simulink model "boundingbox2"  (R2018a)
settings: Solver=VariableStepAuto  StartTime=0.0  StopTime=10.0  RelTol=1e-3
libraries: simulink x127
(part 1 of 4)
settings Model: Creator=Rafael  LastModifiedBy=Rafael

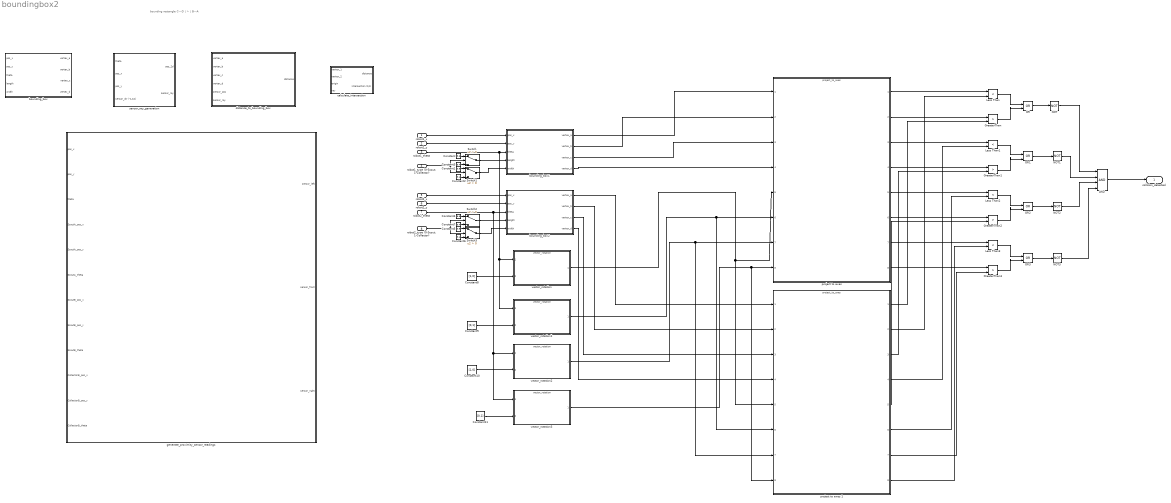
== system boundingbox2 ==
  note: bounding rectangle
      | C---D
      | | > |
      | B---A
  robot1_x : Inport
  robot1_y : Inport  Port=2
  robot1_theta : Inport  Port=3
  robot1_type (0-Scout; 1-Collector) : Inport  Port=4
  robot2_x : Inport  Port=5
  robot2_y : Inport  Port=6
  robot2_theta : Inport  Port=7
  robot2_type (0-Scout; 1-Collector) : Inport  Port=8
  AND : Logic  Inputs=4  IconShape=distinctive  AllPortsSameDT=off  OutDataTypeStr=boolean
  Constant : Constant  Value=8.6
  Constant1 : Constant  Value=9.8
  Constant10 : Constant  Value=[1,0]
  Constant11 : Constant  Value=[0,1]
  Constant{2..3,6..7} (4 alike) : Constant  Value=9.4
  Constant4 : Constant  Value=8.6
  Constant5 : Constant  Value=9.8
  Constant8 : Constant  Value=[1,0]
  Constant9 : Constant  Value=[0,1]
  GreaterThan{,1..3} (4 alike) : RelationalOperator  Operator=>  OutDataTypeStr=boolean  ZeroCross=off  RndMeth=Simplest
  Less Than{,1..3} (4 alike) : RelationalOperator  Operator=<  OutDataTypeStr=boolean  ZeroCross=off  RndMeth=Simplest
  NOT{,1..3} (4 alike) : Logic  Operator=NOT  IconShape=distinctive  AllPortsSameDT=off  OutDataTypeStr=boolean
  OR{,1..3} (4 alike) : Logic  Operator=OR  IconShape=distinctive  AllPortsSameDT=off  OutDataTypeStr=boolean
  Switch{,1..3} (4 alike) : Switch  Criteria=u2 > Threshold  ZeroCross=off
  bounding_box : Subsystem
  bounding_box1 : Subsystem
  bounding_box2 : Subsystem
  "calculate_intersection " : Subsystem
  distance_to_bounding_box : Subsystem
  generate_proximity_sensor_readings : Subsystem
  "project to axes " : ModelReference  ModelNameDialog=project_to_axes  SimulationMode=Normal  ModelReferenceVersion=1.21
  project to axes 1 : ModelReference  ModelNameDialog=project_to_axes  SimulationMode=Normal  ModelReferenceVersion=1.21
  "sensor_ray_generation " : Subsystem
  vector_rotation{,1..3} (4 alike) : ModelReference  ModelNameDialog=vector_rotation  SimulationMode=Normal  ModelReferenceVersion=1.21
  collision_detected : Outport
  wires:
  robot1_x/1 -> bounding_box1/1(pos_x)
  robot1_y/1 -> bounding_box1/2(pos_y)
  robot1_theta/1 -> bounding_box1/3(theta), vector_rotation1/1, vector_rotation/1
  robot1_type (0-Scout; 1-Collector)/1 -> Switch1/2, Switch/2
  Constant/1 -> Switch/1
  Constant1/1 -> Switch1/1
  Constant2/1 -> Switch1/3
  Constant3/1 -> Switch/3
  Switch/1 -> bounding_box1/4(length)
  Switch1/1 -> bounding_box1/5(width)
  robot2_x/1 -> bounding_box2/1(pos_x)
  robot2_y/1 -> bounding_box2/2(pos_y)
  Constant7/1 -> Switch2/3
  Constant6/1 -> Switch3/3
  Constant5/1 -> Switch3/1
  Constant4/1 -> Switch2/1
  robot2_type (0-Scout; 1-Collector)/1 -> Switch2/2, Switch3/2
  Switch2/1 -> bounding_box2/4(length)
  Switch3/1 -> bounding_box2/5(width)
  Constant8/1 -> vector_rotation/2
  Constant9/1 -> vector_rotation1/2
  Constant11/1 -> vector_rotation3/2
  Constant10/1 -> vector_rotation2/2
  robot2_theta/1 -> bounding_box2/3(theta), vector_rotation3/1, vector_rotation2/1
  bounding_box1/1(vertex_a) -> "project to axes "/1
  bounding_box1/2(vertex_b) -> "project to axes "/2
  bounding_box1/3(vertex_c) -> "project to axes "/3
  bounding_box1/4(vertex_d) -> "project to axes "/4
  vector_rotation/1 -> project to axes 1/5, "project to axes "/5
  vector_rotation1/1 -> project to axes 1/6, "project to axes "/6
  vector_rotation2/1 -> project to axes 1/7, "project to axes "/7
  vector_rotation3/1 -> project to axes 1/8, "project to axes "/8
  bounding_box2/1(vertex_a) -> project to axes 1/1
  bounding_box2/2(vertex_b) -> project to axes 1/2
  bounding_box2/3(vertex_c) -> project to axes 1/3
  bounding_box2/4(vertex_d) -> project to axes 1/4
  "project to axes "/1 -> Less Than/1
  project to axes 1/2 -> Less Than/2
  "project to axes "/2 -> GreaterThan/1
  project to axes 1/1 -> GreaterThan/2
  "project to axes "/3 -> Less Than1/1
  project to axes 1/4 -> Less Than1/2
  "project to axes "/4 -> GreaterThan1/1
  project to axes 1/3 -> GreaterThan1/2
  "project to axes "/5 -> Less Than2/1
  project to axes 1/6 -> Less Than2/2
  "project to axes "/6 -> GreaterThan2/1
  "project to axes "/7 -> Less Than3/1
  "project to axes "/8 -> GreaterThan3/1
  project to axes 1/5 -> GreaterThan2/2
  project to axes 1/7 -> GreaterThan3/2
  project to axes 1/8 -> Less Than3/2
  Less Than/1 -> OR/1
  GreaterThan/1 -> OR/2
  Less Than1/1 -> OR1/1
  GreaterThan1/1 -> OR1/2
  Less Than2/1 -> OR2/1
  GreaterThan2/1 -> OR2/2
  Less Than3/1 -> OR3/1
  GreaterThan3/1 -> OR3/2
  OR/1 -> NOT/1
  OR1/1 -> NOT1/1
  OR2/1 -> NOT2/1
  OR3/1 -> NOT3/1
  NOT/1 -> AND/1
  NOT1/1 -> AND/2
  NOT2/1 -> AND/3
  NOT3/1 -> AND/4
  AND/1 -> collision_detected/1

== system boundingbox2/bounding_box ==
  note: output verteces of
      | bounding rectangle
      | C---D
      | |  >  |
      | B---A  as 2d vectors
  pos_x : Inport
  pos_y : Inport  Port=2
  theta : Inport  Port=3
  length : Inport  Port=4
  width : Inport  Port=5
  Add : Sum
  Add1 : Sum
  Gain : Gain  Gain=1/2
  Gain1 : Gain  Gain=1/2
  Gain2 : Gain  Gain=-1
  Subtract : Sum  Inputs=+-
  Subtract1 : Sum  Inputs=+-
  Vector Concatenate : Concatenate
  "vector rotation " : Subsystem
  vector rotation 1 : Subsystem
  vertex_a : Outport
  vertex_b : Outport  Port=2
  vertex_c : Outport  Port=3
  vertex_d : Outport  Port=4
  wires:
  width/1 -> Gain1/1
  length/1 -> Gain/1
  pos_x/1 -> Vector Concatenate/1
  pos_y/1 -> Vector Concatenate/2
  theta/1 -> vector rotation 1/1(angle), "vector rotation "/1(angle)
  Gain/1 -> Gain2/1, "vector rotation "/2(x_dir)
  Gain2/1 -> vector rotation 1/2(x_dir)
  Gain1/1 -> vector rotation 1/3(y_dir), "vector rotation "/3(y_dir)
  Vector Concatenate/1 -> Subtract1/1, Add1/1, Subtract/1, Add/1
  "vector rotation "/1("rotated_vector ") -> Subtract/2, Add/2
  vector rotation 1/1("rotated_vector ") -> Subtract1/2, Add1/2
  Add/1 -> vertex_a/1
  Subtract/1 -> vertex_c/1
  Add1/1 -> vertex_b/1
  Subtract1/1 -> vertex_d/1

== system boundingbox2/bounding_box1 ==
  note: output verteces of
      | bounding rectangle
      | C---D
      | |  >  |
      | B---A  as 2d vectors
  pos_x : Inport
  pos_y : Inport  Port=2
  theta : Inport  Port=3
  length : Inport  Port=4
  width : Inport  Port=5
  Add : Sum
  Add1 : Sum
  Gain : Gain  Gain=1/2
  Gain1 : Gain  Gain=1/2
  Gain2 : Gain  Gain=-1
  Subtract : Sum  Inputs=+-
  Subtract1 : Sum  Inputs=+-
  Vector Concatenate : Concatenate
  "vector rotation " : Subsystem
  vector rotation 1 : Subsystem
  vertex_a : Outport
  vertex_b : Outport  Port=2
  vertex_c : Outport  Port=3
  vertex_d : Outport  Port=4
  wires:
  Subtract1/1 -> vertex_d/1
  Add1/1 -> vertex_b/1
  Subtract/1 -> vertex_c/1
  Add/1 -> vertex_a/1
  vector rotation 1/1("rotated_vector ") -> Add1/2, Subtract1/2
  "vector rotation "/1("rotated_vector ") -> Add/2, Subtract/2
  Vector Concatenate/1 -> Add/1, Subtract/1, Add1/1, Subtract1/1
  Gain1/1 -> "vector rotation "/3(y_dir), vector rotation 1/3(y_dir)
  Gain2/1 -> vector rotation 1/2(x_dir)
  Gain/1 -> "vector rotation "/2(x_dir), Gain2/1
  theta/1 -> "vector rotation "/1(angle), vector rotation 1/1(angle)
  pos_y/1 -> Vector Concatenate/2
  pos_x/1 -> Vector Concatenate/1
  length/1 -> Gain/1
  width/1 -> Gain1/1

== system boundingbox2/bounding_box2 ==
  note: output verteces of
      | bounding rectangle
      | C---D
      | |  >  |
      | B---A  as 2d vectors
  pos_x : Inport
  pos_y : Inport  Port=2
  theta : Inport  Port=3
  length : Inport  Port=4
  width : Inport  Port=5
  Add : Sum
  Add1 : Sum
  Gain : Gain  Gain=1/2
  Gain1 : Gain  Gain=1/2
  Gain2 : Gain  Gain=-1
  Subtract : Sum  Inputs=+-
  Subtract1 : Sum  Inputs=+-
  Vector Concatenate : Concatenate
  "vector rotation " : Subsystem
  vector rotation 1 : Subsystem
  vertex_a : Outport
  vertex_b : Outport  Port=2
  vertex_c : Outport  Port=3
  vertex_d : Outport  Port=4
  wires:
  width/1 -> Gain1/1
  length/1 -> Gain/1
  pos_x/1 -> Vector Concatenate/1
  pos_y/1 -> Vector Concatenate/2
  theta/1 -> vector rotation 1/1(angle), "vector rotation "/1(angle)
  Gain/1 -> Gain2/1, "vector rotation "/2(x_dir)
  Gain2/1 -> vector rotation 1/2(x_dir)
  Gain1/1 -> vector rotation 1/3(y_dir), "vector rotation "/3(y_dir)
  Vector Concatenate/1 -> Subtract1/1, Add1/1, Subtract/1, Add/1
  "vector rotation "/1("rotated_vector ") -> Subtract/2, Add/2
  vector rotation 1/1("rotated_vector ") -> Subtract1/2, Add1/2
  Add/1 -> vertex_a/1
  Subtract/1 -> vertex_c/1
  Add1/1 -> vertex_b/1
  Subtract1/1 -> vertex_d/1

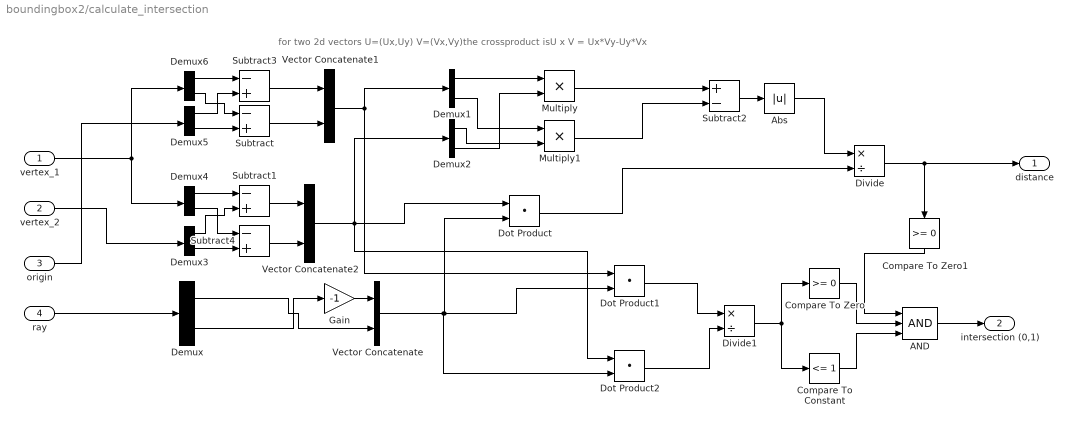
== system boundingbox2/calculate_intersection  ==
  note: for two 2d vectors U=(Ux,Uy) V=(Vx,Vy)the crossproduct isU x V = Ux*Vy-Uy*Vx
  vertex_1 : Inport
  vertex_2 : Inport  Port=2
  "origin " : Inport  Port=3
  ray : Inport  Port=4
  AND : Logic  Inputs=3  IconShape=distinctive  AllPortsSameDT=off  OutDataTypeStr=boolean
  Abs : Abs
  Compare To Constant : simulink/Logic and Bit Operations/Compare To Constant  relop=<=  const=1  OutDataTypeStr=boolean
  Compare To Zero : simulink/Logic and Bit Operations/Compare To Zero  relop=>=  OutDataTypeStr=boolean
  Compare To Zero1 : simulink/Logic and Bit Operations/Compare To Zero  relop=>=  OutDataTypeStr=boolean
  Demux{,1..6} (7 alike) : Demux  Outputs=2
  Divide : Product  Inputs=*/
  Divide1 : Product  Inputs=*/
  Dot Product : DotProduct  InputSameDT=on  OutDataTypeStr=Inherit: Inherit via internal rule
  Dot Product1 : DotProduct  InputSameDT=on  OutDataTypeStr=Inherit: Inherit via internal rule
  Dot Product2 : DotProduct  InputSameDT=on  OutDataTypeStr=Inherit: Inherit via internal rule
  Gain : Gain  Gain=-1
  Multiply : Product
  Multiply1 : Product
  Subtract{,1,3..4} (4 alike) : Sum  Inputs=-+
  Subtract2 : Sum  Inputs=+-
  Vector Concatenate : Concatenate
  Vector Concatenate1 : Concatenate
  Vector Concatenate2 : Concatenate
  distance : Outport
  intersection (0,1) : Outport  Port=2
  wires:
  Compare To Constant/1 -> AND/3
  Compare To Zero/1 -> AND/2
  Divide1/1 -> Compare To Zero/1, Compare To Constant/1
  AND/1 -> intersection (0,1)/1
  Dot Product2/1 -> Divide1/2
  Dot Product1/1 -> Divide1/1
  Multiply1/1 -> Subtract2/2
  Multiply/1 -> Subtract2/1
  Demux2/1 -> Multiply1/2
  Demux1/2 -> Multiply1/1
  Demux2/2 -> Multiply/2
  Demux1/1 -> Multiply/1
  Abs/1 -> Divide/1
  Subtract2/1 -> Abs/1
  Dot Product/1 -> Divide/2
  Divide/1 -> Compare To Zero1/1, distance/1
  Subtract/1 -> Vector Concatenate1/2
  Vector Concatenate/1 -> Dot Product/2, Dot Product1/2, Dot Product2/2
  Demux/1 -> Vector Concatenate/2
  Gain/1 -> Vector Concatenate/1
  Demux/2 -> Gain/1
  ray/1 -> Demux/1
  vertex_2/1 -> Demux3/1
  vertex_1/1 -> Demux6/1, Demux4/1
  "origin "/1 -> Demux5/1
  Demux5/1 -> Subtract3/2
  Demux6/1 -> Subtract3/1
  Demux6/2 -> Subtract/1
  Demux5/2 -> Subtract/2
  Demux4/1 -> Subtract1/1
  Demux4/2 -> Subtract4/1
  Demux3/1 -> Subtract1/2
  Demux3/2 -> Subtract4/2
  Subtract3/1 -> Vector Concatenate1/1
  Vector Concatenate1/1 -> Dot Product1/1, Demux1/1
  Subtract4/1 -> Vector Concatenate2/2
  Subtract1/1 -> Vector Concatenate2/1
  Vector Concatenate2/1 -> Dot Product/1, Demux2/1, Dot Product2/1
  Compare To Zero1/1 -> AND/1

== system boundingbox2/distance_to_bounding_box ==
  note: bounding rectangle
      | C---D
      | |  >  |
      | B---A
  "vertex_a " : Inport
  vertex_b : Inport  Port=2
  vertex_c : Inport  Port=3
  vertex_d : Inport  Port=4
  sensor_pos : Inport  Port=5
  "sensor_ray " : Inport  Port=6
  Inf{,1..3} (4 alike) : Constant  Value=inf
  Min : MinMax  Inputs=4
  Switch{,1..3} (4 alike) : Switch  Criteria=u2 > Threshold
  "calculate_intersection " : Subsystem
  calculate_intersection 1 : Subsystem
  calculate_intersection 2 : Subsystem
  calculate_intersection 3 : Subsystem
  distance : Outport
  wires:
  "vertex_a "/1 -> calculate_intersection 3/2(vertex_2), "calculate_intersection "/1(vertex_1)
  vertex_b/1 -> calculate_intersection 1/1(vertex_1), "calculate_intersection "/2(vertex_2)
  vertex_c/1 -> calculate_intersection 2/1(vertex_1), calculate_intersection 1/2(vertex_2)
  vertex_d/1 -> calculate_intersection 3/1(vertex_1), calculate_intersection 2/2(vertex_2)
  sensor_pos/1 -> calculate_intersection 3/3("origin "), calculate_intersection 2/3("origin "), calculate_intersection 1/3("origin "), "calculate_intersection "/3("origin ")
  "sensor_ray "/1 -> calculate_intersection 3/4(ray), calculate_intersection 2/4(ray), calculate_intersection 1/4(ray), "calculate_intersection "/4(ray)
  "calculate_intersection "/2(intersection (0,1)) -> Switch/2
  Inf/1 -> Switch/3
  Inf1/1 -> Switch1/3
  calculate_intersection 1/2(intersection (0,1)) -> Switch1/2
  calculate_intersection 2/2(intersection (0,1)) -> Switch2/2
  calculate_intersection 3/2(intersection (0,1)) -> Switch3/2
  Inf2/1 -> Switch2/3
  Inf3/1 -> Switch3/3
  calculate_intersection 3/1(distance) -> Switch3/1
  calculate_intersection 2/1(distance) -> Switch2/1
  calculate_intersection 1/1(distance) -> Switch1/1
  "calculate_intersection "/1(distance) -> Switch/1
  Switch/1 -> Min/1
  Switch1/1 -> Min/2
  Switch2/1 -> Min/3
  Switch3/1 -> Min/4
  Min/1 -> distance/1

== system boundingbox2/generate_proximity_sensor_readings ==
  pos_x : Inport
  pos_y : Inport  Port=2
  theta : Inport  Port=3
  ScoutA_pos_x : Inport  Port=4
  ScoutA_pos_y : Inport  Port=5
  ScoutA_theta : Inport  Port=6
  ScoutB_pos_x : Inport  Port=7
  ScoutB_pos_y : Inport  Port=8
  ScoutB_theta : Inport  Port=9
  CollectorB_pos_x : Inport  Port=10
  CollectorB_pos_y : Inport  Port=11
  CollectorB_theta : Inport  Port=12
  Constant{,4..6} (4 alike) : Constant  Value=9.4
  Constant1 : Constant  Value=-1
  Constant2 : Constant  Value=0
  Constant3 : Constant
  Constant7 : Constant  Value=8.6
  Constant8 : Constant  Value=9.8
  Subsystem : Subsystem
  Subsystem1 : Subsystem
  Subsystem2 : Subsystem
  bounding_box_CollectorB : Subsystem
  bounding_box_ScoutA : Subsystem
  bounding_box_ScoutB : Subsystem
  sensor_ray_generation front : Subsystem
  sensor_ray_generation left : Subsystem
  sensor_ray_generation right : Subsystem
  sensor_left : Outport
  sensor_front : Outport  Port=2
  "sensor_right " : Outport  Port=3
  wires:
  theta/1 -> sensor_ray_generation right/1("theta "), sensor_ray_generation front/1("theta "), sensor_ray_generation left/1("theta ")
  bounding_box_CollectorB/2(vertex_b) -> Subsystem2/14(CollectorB_b), Subsystem1/14(CollectorB_b), Subsystem/14(CollectorB_b)
  Constant2/1 -> sensor_ray_generation front/4("sensor_dir (-1,0,1) ")
  Subsystem2/1("sensor_data ") -> "sensor_right "/1
  bounding_box_ScoutB/4(vertex_d) -> Subsystem2/8(ScoutB_d), Subsystem1/8(ScoutB_d), Subsystem/8(ScoutB_d)
  Constant8/1 -> bounding_box_CollectorB/5(width)
  bounding_box_ScoutA/1(vertex_a) -> Subsystem2/5(ScoutA_a), Subsystem1/5(ScoutA_a), Subsystem/5(ScoutA_a)
  bounding_box_CollectorB/3(vertex_c) -> Subsystem2/11(CollectorB_c), Subsystem1/11(CollectorB_c), Subsystem/11(CollectorB_c)
  ScoutB_theta/1 -> bounding_box_ScoutB/3(theta)
  Constant5/1 -> bounding_box_ScoutB/4(length)
  ScoutA_pos_x/1 -> bounding_box_ScoutA/1(pos_x)
  bounding_box_ScoutA/3(vertex_c) -> Subsystem2/3(ScoutA_c), Subsystem1/3(ScoutA_c), Subsystem/3(ScoutA_c)
  Constant6/1 -> bounding_box_ScoutB/5(width)
  Constant1/1 -> sensor_ray_generation left/4("sensor_dir (-1,0,1) ")
  bounding_box_CollectorB/1(vertex_a) -> Subsystem2/13(CollectorB_a), Subsystem1/13(CollectorB_a), Subsystem/13(CollectorB_a)
  bounding_box_ScoutA/4(vertex_d) -> Subsystem2/4(ScoutA_d), Subsystem1/4(ScoutA_d), Subsystem/4(ScoutA_d)
  sensor_ray_generation front/1(pos_2d) -> Subsystem1/1(origin_pos)
  sensor_ray_generation left/2("sensor_ray ") -> Subsystem/2(sensor_ray_dir)
  bounding_box_CollectorB/4(vertex_d) -> Subsystem2/12(CollectorB_d), Subsystem1/12(CollectorB_d), Subsystem/12(CollectorB_d)
  ScoutB_pos_y/1 -> bounding_box_ScoutB/2(pos_y)
  Subsystem/1("sensor_data ") -> sensor_left/1
  pos_y/1 -> sensor_ray_generation left/3(pos_y)
  bounding_box_ScoutB/2(vertex_b) -> Subsystem2/10(ScoutB_b), Subsystem/10(ScoutB_b), Subsystem1/10(ScoutB_b)
  Subsystem1/1("sensor_data ") -> sensor_front/1
  bounding_box_ScoutB/1(vertex_a) -> Subsystem2/9(ScoutB_a), Subsystem1/9(ScoutB_a), Subsystem/9(ScoutB_a)
  bounding_box_ScoutA/2(vertex_b) -> Subsystem2/6(ScoutA_b), Subsystem1/6(ScoutA_b), Subsystem/6(ScoutA_b)
  bounding_box_ScoutB/3(vertex_c) -> Subsystem2/7(ScoutB_c), Subsystem1/7(ScoutB_c), Subsystem/7(ScoutB_c)
  sensor_ray_generation right/2("sensor_ray ") -> Subsystem2/2(sensor_ray_dir)
  ScoutA_pos_y/1 -> bounding_box_ScoutA/2(pos_y)
  CollectorB_theta/1 -> bounding_box_CollectorB/3(theta)
  pos_x/1 -> sensor_ray_generation right/3(pos_y), sensor_ray_generation front/3(pos_y), sensor_ray_generation right/2(pos_x), sensor_ray_generation front/2(pos_x), sensor_ray_generation left/2(pos_x)
  sensor_ray_generation right/1(pos_2d) -> Subsystem2/1(origin_pos)
  Constant4/1 -> bounding_box_ScoutA/5(width)
  CollectorB_pos_x/1 -> bounding_box_CollectorB/1(pos_x)
  Constant/1 -> bounding_box_ScoutA/4(length)
  CollectorB_pos_y/1 -> bounding_box_CollectorB/2(pos_y)
  Constant7/1 -> bounding_box_CollectorB/4(length)
  ScoutA_theta/1 -> bounding_box_ScoutA/3(theta)
  ScoutB_pos_x/1 -> bounding_box_ScoutB/1(pos_x)
  Constant3/1 -> sensor_ray_generation right/4("sensor_dir (-1,0,1) ")
  sensor_ray_generation left/1(pos_2d) -> Subsystem/1(origin_pos)
  sensor_ray_generation front/2("sensor_ray ") -> Subsystem1/2(sensor_ray_dir)

== system boundingbox2/sensor_ray_generation  ==
  "theta " : Inport
  pos_x : Inport  Port=2
  pos_y : Inport  Port=3
  "sensor_dir (-1,0,1) " : Inport  Port=4
  Compare To Zero : simulink/Logic and Bit Operations/Compare To Zero  relop===  OutDataTypeStr=boolean
  Constant : Constant  Value=1.0
  Constant1 : Constant  Value=0
  Switch : Switch  Threshold=1
  Vector Concatenate : Concatenate
  "vector rotation " : Subsystem
  pos_2d : Outport
  "sensor_ray " : Outport  Port=2
  wires:
  "vector rotation "/1("rotated_vector ") -> "sensor_ray "/1
  pos_y/1 -> Vector Concatenate/2
  Vector Concatenate/1 -> pos_2d/1
  pos_x/1 -> Vector Concatenate/1
  "sensor_dir (-1,0,1) "/1 -> Compare To Zero/1, "vector rotation "/3(y_dir)
  "theta "/1 -> "vector rotation "/1(angle)
  Compare To Zero/1 -> Switch/2
  Constant/1 -> Switch/1
  Constant1/1 -> Switch/3
  Switch/1 -> "vector rotation "/2(x_dir)

== system boundingbox2/bounding_box/vector rotation  ==
  angle : Inport
  x_dir : Inport  Port=2
  y_dir : Inport  Port=3
  Cos : Trigonometry  Operator=cos
  Multiply{,1..3} (4 alike) : Product
  Sin : Trigonometry
  Subtract : Sum  Inputs=+-
  Subtract1 : Sum
  Vector Concatenate1 : Concatenate
  "rotated_vector " : Outport
  wires:
  Multiply3/1 -> Subtract1/2
  Multiply1/1 -> Subtract1/1
  Multiply/1 -> Subtract/1
  y_dir/1 -> Multiply3/1, Multiply2/1
  Subtract1/1 -> Vector Concatenate1/2
  Cos/1 -> Multiply3/2, Multiply/2
  Sin/1 -> Multiply1/2, Multiply2/2
  angle/1 -> Cos/1, Sin/1
  x_dir/1 -> Multiply1/1, Multiply/1
  Vector Concatenate1/1 -> "rotated_vector "/1
  Subtract/1 -> Vector Concatenate1/1
  Multiply2/1 -> Subtract/2

== system boundingbox2/bounding_box/vector rotation 1 ==
  angle : Inport
  x_dir : Inport  Port=2
  y_dir : Inport  Port=3
  Cos : Trigonometry  Operator=cos
  Multiply{,1..3} (4 alike) : Product
  Sin : Trigonometry
  Subtract : Sum  Inputs=+-
  Subtract1 : Sum
  Vector Concatenate1 : Concatenate
  "rotated_vector " : Outport
  wires:
  Multiply2/1 -> Subtract/2
  Subtract/1 -> Vector Concatenate1/1
  Vector Concatenate1/1 -> "rotated_vector "/1
  x_dir/1 -> Multiply/1, Multiply1/1
  angle/1 -> Sin/1, Cos/1
  Sin/1 -> Multiply2/2, Multiply1/2
  Cos/1 -> Multiply/2, Multiply3/2
  Subtract1/1 -> Vector Concatenate1/2
  y_dir/1 -> Multiply2/1, Multiply3/1
  Multiply/1 -> Subtract/1
  Multiply1/1 -> Subtract1/1
  Multiply3/1 -> Subtract1/2

== system boundingbox2/bounding_box1/vector rotation  ==
  angle : Inport
  x_dir : Inport  Port=2
  y_dir : Inport  Port=3
  Cos : Trigonometry  Operator=cos
  Multiply{,1..3} (4 alike) : Product
  Sin : Trigonometry
  Subtract : Sum  Inputs=+-
  Subtract1 : Sum
  Vector Concatenate1 : Concatenate
  "rotated_vector " : Outport
  wires:
  Multiply2/1 -> Subtract/2
  Subtract/1 -> Vector Concatenate1/1
  Vector Concatenate1/1 -> "rotated_vector "/1
  x_dir/1 -> Multiply/1, Multiply1/1
  angle/1 -> Sin/1, Cos/1
  Sin/1 -> Multiply2/2, Multiply1/2
  Cos/1 -> Multiply/2, Multiply3/2
  Subtract1/1 -> Vector Concatenate1/2
  y_dir/1 -> Multiply2/1, Multiply3/1
  Multiply/1 -> Subtract/1
  Multiply1/1 -> Subtract1/1
  Multiply3/1 -> Subtract1/2

== system boundingbox2/bounding_box1/vector rotation 1 ==
  angle : Inport
  x_dir : Inport  Port=2
  y_dir : Inport  Port=3
  Cos : Trigonometry  Operator=cos
  Multiply{,1..3} (4 alike) : Product
  Sin : Trigonometry
  Subtract : Sum  Inputs=+-
  Subtract1 : Sum
  Vector Concatenate1 : Concatenate
  "rotated_vector " : Outport
  wires:
  Multiply3/1 -> Subtract1/2
  Multiply1/1 -> Subtract1/1
  Multiply/1 -> Subtract/1
  y_dir/1 -> Multiply3/1, Multiply2/1
  Subtract1/1 -> Vector Concatenate1/2
  Cos/1 -> Multiply3/2, Multiply/2
  Sin/1 -> Multiply1/2, Multiply2/2
  angle/1 -> Cos/1, Sin/1
  x_dir/1 -> Multiply1/1, Multiply/1
  Vector Concatenate1/1 -> "rotated_vector "/1
  Subtract/1 -> Vector Concatenate1/1
  Multiply2/1 -> Subtract/2

== system boundingbox2/bounding_box2/vector rotation  ==
  angle : Inport
  x_dir : Inport  Port=2
  y_dir : Inport  Port=3
  Cos : Trigonometry  Operator=cos
  Multiply{,1..3} (4 alike) : Product
  Sin : Trigonometry
  Subtract : Sum  Inputs=+-
  Subtract1 : Sum
  Vector Concatenate1 : Concatenate
  "rotated_vector " : Outport
  wires:
  Multiply3/1 -> Subtract1/2
  Multiply1/1 -> Subtract1/1
  Multiply/1 -> Subtract/1
  y_dir/1 -> Multiply3/1, Multiply2/1
  Subtract1/1 -> Vector Concatenate1/2
  Cos/1 -> Multiply3/2, Multiply/2
  Sin/1 -> Multiply1/2, Multiply2/2
  angle/1 -> Cos/1, Sin/1
  x_dir/1 -> Multiply1/1, Multiply/1
  Vector Concatenate1/1 -> "rotated_vector "/1
  Subtract/1 -> Vector Concatenate1/1
  Multiply2/1 -> Subtract/2

== system boundingbox2/bounding_box2/vector rotation 1 ==
  angle : Inport
  x_dir : Inport  Port=2
  y_dir : Inport  Port=3
  Cos : Trigonometry  Operator=cos
  Multiply{,1..3} (4 alike) : Product
  Sin : Trigonometry
  Subtract : Sum  Inputs=+-
  Subtract1 : Sum
  Vector Concatenate1 : Concatenate
  "rotated_vector " : Outport
  wires:
  Multiply2/1 -> Subtract/2
  Subtract/1 -> Vector Concatenate1/1
  Vector Concatenate1/1 -> "rotated_vector "/1
  x_dir/1 -> Multiply/1, Multiply1/1
  angle/1 -> Sin/1, Cos/1
  Sin/1 -> Multiply2/2, Multiply1/2
  Cos/1 -> Multiply/2, Multiply3/2
  Subtract1/1 -> Vector Concatenate1/2
  y_dir/1 -> Multiply2/1, Multiply3/1
  Multiply/1 -> Subtract/1
  Multiply1/1 -> Subtract1/1
  Multiply3/1 -> Subtract1/2

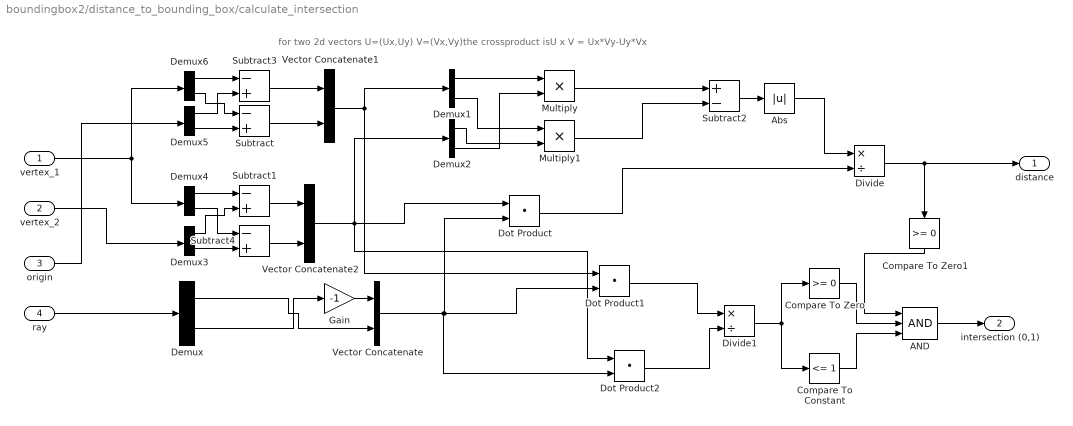
== system boundingbox2/distance_to_bounding_box/calculate_intersection  ==
  note: for two 2d vectors U=(Ux,Uy) V=(Vx,Vy)the crossproduct isU x V = Ux*Vy-Uy*Vx
  vertex_1 : Inport
  vertex_2 : Inport  Port=2
  "origin " : Inport  Port=3
  ray : Inport  Port=4
  AND : Logic  Inputs=3  IconShape=distinctive  AllPortsSameDT=off  OutDataTypeStr=boolean
  Abs : Abs
  Compare To Constant : simulink/Logic and Bit Operations/Compare To Constant  relop=<=  const=1  OutDataTypeStr=boolean
  Compare To Zero : simulink/Logic and Bit Operations/Compare To Zero  relop=>=  OutDataTypeStr=boolean
  Compare To Zero1 : simulink/Logic and Bit Operations/Compare To Zero  relop=>=  OutDataTypeStr=boolean
  Demux{,1..6} (7 alike) : Demux  Outputs=2
  Divide : Product  Inputs=*/
  Divide1 : Product  Inputs=*/
  Dot Product : DotProduct  InputSameDT=on  OutDataTypeStr=Inherit: Inherit via internal rule
  Dot Product1 : DotProduct  InputSameDT=on  OutDataTypeStr=Inherit: Inherit via internal rule
  Dot Product2 : DotProduct  InputSameDT=on  OutDataTypeStr=Inherit: Inherit via internal rule
  Gain : Gain  Gain=-1
  Multiply : Product
  Multiply1 : Product
  Subtract{,1,3..4} (4 alike) : Sum  Inputs=-+
  Subtract2 : Sum  Inputs=+-
  Vector Concatenate : Concatenate
  Vector Concatenate1 : Concatenate
  Vector Concatenate2 : Concatenate
  distance : Outport
  intersection (0,1) : Outport  Port=2
  wires:
  Compare To Constant/1 -> AND/3
  Compare To Zero/1 -> AND/2
  Divide1/1 -> Compare To Zero/1, Compare To Constant/1
  AND/1 -> intersection (0,1)/1
  Dot Product2/1 -> Divide1/2
  Dot Product1/1 -> Divide1/1
  Multiply1/1 -> Subtract2/2
  Multiply/1 -> Subtract2/1
  Demux2/1 -> Multiply1/2
  Demux1/2 -> Multiply1/1
  Demux2/2 -> Multiply/2
  Demux1/1 -> Multiply/1
  Abs/1 -> Divide/1
  Subtract2/1 -> Abs/1
  Dot Product/1 -> Divide/2
  Divide/1 -> Compare To Zero1/1, distance/1
  Subtract/1 -> Vector Concatenate1/2
  Vector Concatenate/1 -> Dot Product/2, Dot Product1/2, Dot Product2/2
  Demux/1 -> Vector Concatenate/2
  Gain/1 -> Vector Concatenate/1
  Demux/2 -> Gain/1
  ray/1 -> Demux/1
  vertex_2/1 -> Demux3/1
  vertex_1/1 -> Demux6/1, Demux4/1
  "origin "/1 -> Demux5/1
  Demux5/1 -> Subtract3/2
  Demux6/1 -> Subtract3/1
  Demux6/2 -> Subtract/1
  Demux5/2 -> Subtract/2
  Demux4/1 -> Subtract1/1
  Demux4/2 -> Subtract4/1
  Demux3/1 -> Subtract1/2
  Demux3/2 -> Subtract4/2
  Subtract3/1 -> Vector Concatenate1/1
  Vector Concatenate1/1 -> Dot Product1/1, Demux1/1
  Subtract4/1 -> Vector Concatenate2/2
  Subtract1/1 -> Vector Concatenate2/1
  Vector Concatenate2/1 -> Dot Product/1, Demux2/1, Dot Product2/1
  Compare To Zero1/1 -> AND/1

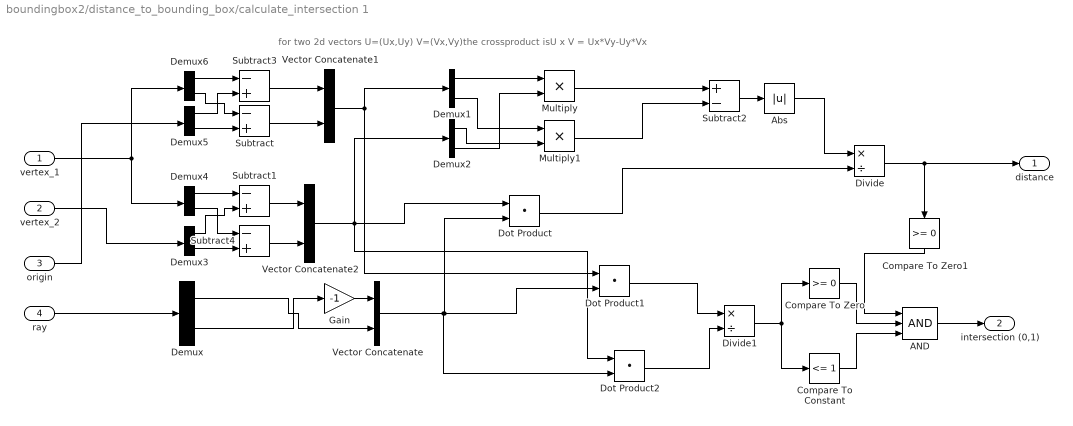
== system boundingbox2/distance_to_bounding_box/calculate_intersection 1 ==
  note: for two 2d vectors U=(Ux,Uy) V=(Vx,Vy)the crossproduct isU x V = Ux*Vy-Uy*Vx
  vertex_1 : Inport
  vertex_2 : Inport  Port=2
  "origin " : Inport  Port=3
  ray : Inport  Port=4
  AND : Logic  Inputs=3  IconShape=distinctive  AllPortsSameDT=off  OutDataTypeStr=boolean
  Abs : Abs
  Compare To Constant : simulink/Logic and Bit Operations/Compare To Constant  relop=<=  const=1  OutDataTypeStr=boolean
  Compare To Zero : simulink/Logic and Bit Operations/Compare To Zero  relop=>=  OutDataTypeStr=boolean
  Compare To Zero1 : simulink/Logic and Bit Operations/Compare To Zero  relop=>=  OutDataTypeStr=boolean
  Demux{,1..6} (7 alike) : Demux  Outputs=2
  Divide : Product  Inputs=*/
  Divide1 : Product  Inputs=*/
  Dot Product : DotProduct  InputSameDT=on  OutDataTypeStr=Inherit: Inherit via internal rule
  Dot Product1 : DotProduct  InputSameDT=on  OutDataTypeStr=Inherit: Inherit via internal rule
  Dot Product2 : DotProduct  InputSameDT=on  OutDataTypeStr=Inherit: Inherit via internal rule
  Gain : Gain  Gain=-1
  Multiply : Product
  Multiply1 : Product
  Subtract{,1,3..4} (4 alike) : Sum  Inputs=-+
  Subtract2 : Sum  Inputs=+-
  Vector Concatenate : Concatenate
  Vector Concatenate1 : Concatenate
  Vector Concatenate2 : Concatenate
  distance : Outport
  intersection (0,1) : Outport  Port=2
  wires:
  Compare To Zero1/1 -> AND/1
  Vector Concatenate2/1 -> Dot Product2/1, Demux2/1, Dot Product/1
  Subtract1/1 -> Vector Concatenate2/1
  Subtract4/1 -> Vector Concatenate2/2
  Vector Concatenate1/1 -> Demux1/1, Dot Product1/1
  Subtract3/1 -> Vector Concatenate1/1
  Demux3/2 -> Subtract4/2
  Demux3/1 -> Subtract1/2
  Demux4/2 -> Subtract4/1
  Demux4/1 -> Subtract1/1
  Demux5/2 -> Subtract/2
  Demux6/2 -> Subtract/1
  Demux6/1 -> Subtract3/1
  Demux5/1 -> Subtract3/2
  "origin "/1 -> Demux5/1
  vertex_1/1 -> Demux4/1, Demux6/1
  vertex_2/1 -> Demux3/1
  ray/1 -> Demux/1
  Demux/2 -> Gain/1
  Gain/1 -> Vector Concatenate/1
  Demux/1 -> Vector Concatenate/2
  Vector Concatenate/1 -> Dot Product2/2, Dot Product1/2, Dot Product/2
  Subtract/1 -> Vector Concatenate1/2
  Divide/1 -> distance/1, Compare To Zero1/1
  Dot Product/1 -> Divide/2
  Subtract2/1 -> Abs/1
  Abs/1 -> Divide/1
  Demux1/1 -> Multiply/1
  Demux2/2 -> Multiply/2
  Demux1/2 -> Multiply1/1
  Demux2/1 -> Multiply1/2
  Multiply/1 -> Subtract2/1
  Multiply1/1 -> Subtract2/2
  Dot Product1/1 -> Divide1/1
  Dot Product2/1 -> Divide1/2
  AND/1 -> intersection (0,1)/1
  Divide1/1 -> Compare To Constant/1, Compare To Zero/1
  Compare To Zero/1 -> AND/2
  Compare To Constant/1 -> AND/3

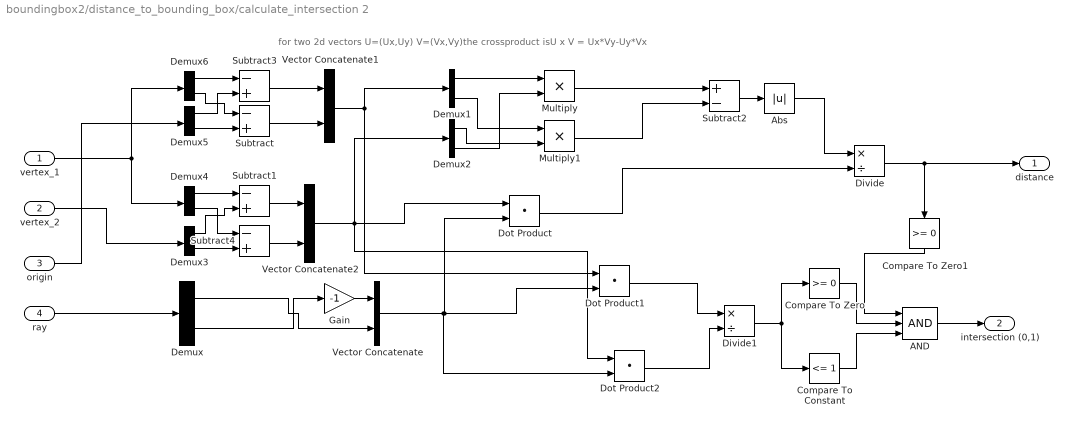
== system boundingbox2/distance_to_bounding_box/calculate_intersection 2 ==
  note: for two 2d vectors U=(Ux,Uy) V=(Vx,Vy)the crossproduct isU x V = Ux*Vy-Uy*Vx
  vertex_1 : Inport
  vertex_2 : Inport  Port=2
  "origin " : Inport  Port=3
  ray : Inport  Port=4
  AND : Logic  Inputs=3  IconShape=distinctive  AllPortsSameDT=off  OutDataTypeStr=boolean
  Abs : Abs
  Compare To Constant : simulink/Logic and Bit Operations/Compare To Constant  relop=<=  const=1  OutDataTypeStr=boolean
  Compare To Zero : simulink/Logic and Bit Operations/Compare To Zero  relop=>=  OutDataTypeStr=boolean
  Compare To Zero1 : simulink/Logic and Bit Operations/Compare To Zero  relop=>=  OutDataTypeStr=boolean
  Demux{,1..6} (7 alike) : Demux  Outputs=2
  Divide : Product  Inputs=*/
  Divide1 : Product  Inputs=*/
  Dot Product : DotProduct  InputSameDT=on  OutDataTypeStr=Inherit: Inherit via internal rule
  Dot Product1 : DotProduct  InputSameDT=on  OutDataTypeStr=Inherit: Inherit via internal rule
  Dot Product2 : DotProduct  InputSameDT=on  OutDataTypeStr=Inherit: Inherit via internal rule
  Gain : Gain  Gain=-1
  Multiply : Product
  Multiply1 : Product
  Subtract{,1,3..4} (4 alike) : Sum  Inputs=-+
  Subtract2 : Sum  Inputs=+-
  Vector Concatenate : Concatenate
  Vector Concatenate1 : Concatenate
  Vector Concatenate2 : Concatenate
  distance : Outport
  intersection (0,1) : Outport  Port=2
  wires:
  Compare To Constant/1 -> AND/3
  Compare To Zero/1 -> AND/2
  Divide1/1 -> Compare To Zero/1, Compare To Constant/1
  AND/1 -> intersection (0,1)/1
  Dot Product2/1 -> Divide1/2
  Dot Product1/1 -> Divide1/1
  Multiply1/1 -> Subtract2/2
  Multiply/1 -> Subtract2/1
  Demux2/1 -> Multiply1/2
  Demux1/2 -> Multiply1/1
  Demux2/2 -> Multiply/2
  Demux1/1 -> Multiply/1
  Abs/1 -> Divide/1
  Subtract2/1 -> Abs/1
  Dot Product/1 -> Divide/2
  Divide/1 -> Compare To Zero1/1, distance/1
  Subtract/1 -> Vector Concatenate1/2
  Vector Concatenate/1 -> Dot Product/2, Dot Product1/2, Dot Product2/2
  Demux/1 -> Vector Concatenate/2
  Gain/1 -> Vector Concatenate/1
  Demux/2 -> Gain/1
  ray/1 -> Demux/1
  vertex_2/1 -> Demux3/1
  vertex_1/1 -> Demux6/1, Demux4/1
  "origin "/1 -> Demux5/1
  Demux5/1 -> Subtract3/2
  Demux6/1 -> Subtract3/1
  Demux6/2 -> Subtract/1
  Demux5/2 -> Subtract/2
  Demux4/1 -> Subtract1/1
  Demux4/2 -> Subtract4/1
  Demux3/1 -> Subtract1/2
  Demux3/2 -> Subtract4/2
  Subtract3/1 -> Vector Concatenate1/1
  Vector Concatenate1/1 -> Dot Product1/1, Demux1/1
  Subtract4/1 -> Vector Concatenate2/2
  Subtract1/1 -> Vector Concatenate2/1
  Vector Concatenate2/1 -> Dot Product/1, Demux2/1, Dot Product2/1
  Compare To Zero1/1 -> AND/1

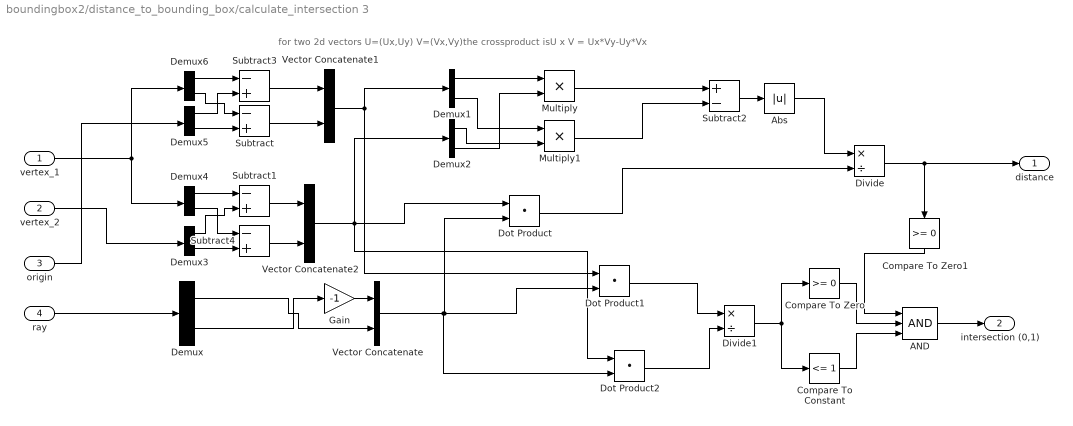
== system boundingbox2/distance_to_bounding_box/calculate_intersection 3 ==
  note: for two 2d vectors U=(Ux,Uy) V=(Vx,Vy)the crossproduct isU x V = Ux*Vy-Uy*Vx
  vertex_1 : Inport
  vertex_2 : Inport  Port=2
  "origin " : Inport  Port=3
  ray : Inport  Port=4
  AND : Logic  Inputs=3  IconShape=distinctive  AllPortsSameDT=off  OutDataTypeStr=boolean
  Abs : Abs
  Compare To Constant : simulink/Logic and Bit Operations/Compare To Constant  relop=<=  const=1  OutDataTypeStr=boolean
  Compare To Zero : simulink/Logic and Bit Operations/Compare To Zero  relop=>=  OutDataTypeStr=boolean
  Compare To Zero1 : simulink/Logic and Bit Operations/Compare To Zero  relop=>=  OutDataTypeStr=boolean
  Demux{,1..6} (7 alike) : Demux  Outputs=2
  Divide : Product  Inputs=*/
  Divide1 : Product  Inputs=*/
  Dot Product : DotProduct  InputSameDT=on  OutDataTypeStr=Inherit: Inherit via internal rule
  Dot Product1 : DotProduct  InputSameDT=on  OutDataTypeStr=Inherit: Inherit via internal rule
  Dot Product2 : DotProduct  InputSameDT=on  OutDataTypeStr=Inherit: Inherit via internal rule
  Gain : Gain  Gain=-1
  Multiply : Product
  Multiply1 : Product
  Subtract{,1,3..4} (4 alike) : Sum  Inputs=-+
  Subtract2 : Sum  Inputs=+-
  Vector Concatenate : Concatenate
  Vector Concatenate1 : Concatenate
  Vector Concatenate2 : Concatenate
  distance : Outport
  intersection (0,1) : Outport  Port=2
  wires:
  Compare To Zero1/1 -> AND/1
  Vector Concatenate2/1 -> Dot Product2/1, Demux2/1, Dot Product/1
  Subtract1/1 -> Vector Concatenate2/1
  Subtract4/1 -> Vector Concatenate2/2
  Vector Concatenate1/1 -> Demux1/1, Dot Product1/1
  Subtract3/1 -> Vector Concatenate1/1
  Demux3/2 -> Subtract4/2
  Demux3/1 -> Subtract1/2
  Demux4/2 -> Subtract4/1
  Demux4/1 -> Subtract1/1
  Demux5/2 -> Subtract/2
  Demux6/2 -> Subtract/1
  Demux6/1 -> Subtract3/1
  Demux5/1 -> Subtract3/2
  "origin "/1 -> Demux5/1
  vertex_1/1 -> Demux4/1, Demux6/1
  vertex_2/1 -> Demux3/1
  ray/1 -> Demux/1
  Demux/2 -> Gain/1
  Gain/1 -> Vector Concatenate/1
  Demux/1 -> Vector Concatenate/2
  Vector Concatenate/1 -> Dot Product2/2, Dot Product1/2, Dot Product/2
  Subtract/1 -> Vector Concatenate1/2
  Divide/1 -> distance/1, Compare To Zero1/1
  Dot Product/1 -> Divide/2
  Subtract2/1 -> Abs/1
  Abs/1 -> Divide/1
  Demux1/1 -> Multiply/1
  Demux2/2 -> Multiply/2
  Demux1/2 -> Multiply1/1
  Demux2/1 -> Multiply1/2
  Multiply/1 -> Subtract2/1
  Multiply1/1 -> Subtract2/2
  Dot Product1/1 -> Divide1/1
  Dot Product2/1 -> Divide1/2
  AND/1 -> intersection (0,1)/1
  Divide1/1 -> Compare To Constant/1, Compare To Zero/1
  Compare To Zero/1 -> AND/2
  Compare To Constant/1 -> AND/3

== system boundingbox2/generate_proximity_sensor_readings/Subsystem ==
  origin_pos : Inport
  sensor_ray_dir : Inport  Port=2
  ScoutA_c : Inport  Port=3
  ScoutA_d : Inport  Port=4
  ScoutA_a : Inport  Port=5
  ScoutA_b : Inport  Port=6
  ScoutB_c : Inport  Port=7
  ScoutB_d : Inport  Port=8
  ScoutB_a : Inport  Port=9
  ScoutB_b : Inport  Port=10
  CollectorB_c : Inport  Port=11
  CollectorB_d : Inport  Port=12
  CollectorB_a : Inport  Port=13
  CollectorB_b : Inport  Port=14
  Min : MinMax  Inputs=3
  distance_to_bounding_box : Subsystem
  distance_to_bounding_box1 : Subsystem
  distance_to_bounding_box2 : Subsystem
  "distance_to_proximity_sensor_data " : Subsystem
  "sensor_data " : Outport
  wires:
  distance_to_bounding_box/1(distance) -> Min/1
  sensor_ray_dir/1 -> distance_to_bounding_box/6("sensor_ray "), distance_to_bounding_box1/6("sensor_ray "), distance_to_bounding_box2/6("sensor_ray ")
  Min/1 -> "distance_to_proximity_sensor_data "/1(distance_cm)
  origin_pos/1 -> distance_to_bounding_box/5(sensor_pos), distance_to_bounding_box1/5(sensor_pos), distance_to_bounding_box2/5(sensor_pos)
  ScoutA_c/1 -> distance_to_bounding_box/3(vertex_c)
  ScoutA_b/1 -> distance_to_bounding_box/2(vertex_b)
  CollectorB_c/1 -> distance_to_bounding_box2/3(vertex_c)
  ScoutA_d/1 -> distance_to_bounding_box/4(vertex_d)
  ScoutB_c/1 -> distance_to_bounding_box1/3(vertex_c)
  ScoutA_a/1 -> distance_to_bounding_box/1("vertex_a ")
  ScoutB_d/1 -> distance_to_bounding_box1/4(vertex_d)
  distance_to_bounding_box2/1(distance) -> Min/3
  ScoutB_b/1 -> distance_to_bounding_box1/2(vertex_b)
  ScoutB_a/1 -> distance_to_bounding_box1/1("vertex_a ")
  CollectorB_a/1 -> distance_to_bounding_box2/1("vertex_a ")
  CollectorB_d/1 -> distance_to_bounding_box2/4(vertex_d)
  distance_to_bounding_box1/1(distance) -> Min/2
  CollectorB_b/1 -> distance_to_bounding_box2/2(vertex_b)
  "distance_to_proximity_sensor_data "/1("prox_sensor_input ") -> "sensor_data "/1

== system boundingbox2/generate_proximity_sensor_readings/Subsystem1 ==
  origin_pos : Inport
  sensor_ray_dir : Inport  Port=2
  ScoutA_c : Inport  Port=3
  ScoutA_d : Inport  Port=4
  ScoutA_a : Inport  Port=5
  ScoutA_b : Inport  Port=6
  ScoutB_c : Inport  Port=7
  ScoutB_d : Inport  Port=8
  ScoutB_a : Inport  Port=9
  ScoutB_b : Inport  Port=10
  CollectorB_c : Inport  Port=11
  CollectorB_d : Inport  Port=12
  CollectorB_a : Inport  Port=13
  CollectorB_b : Inport  Port=14
  Min : MinMax  Inputs=3
  distance_to_bounding_box : Subsystem
  distance_to_bounding_box1 : Subsystem
  distance_to_bounding_box2 : Subsystem
  "distance_to_proximity_sensor_data " : Subsystem
  "sensor_data " : Outport
  wires:
  "distance_to_proximity_sensor_data "/1("prox_sensor_input ") -> "sensor_data "/1
  CollectorB_b/1 -> distance_to_bounding_box2/2(vertex_b)
  distance_to_bounding_box1/1(distance) -> Min/2
  CollectorB_d/1 -> distance_to_bounding_box2/4(vertex_d)
  CollectorB_a/1 -> distance_to_bounding_box2/1("vertex_a ")
  ScoutB_a/1 -> distance_to_bounding_box1/1("vertex_a ")
  ScoutB_b/1 -> distance_to_bounding_box1/2(vertex_b)
  distance_to_bounding_box2/1(distance) -> Min/3
  ScoutB_d/1 -> distance_to_bounding_box1/4(vertex_d)
  ScoutA_a/1 -> distance_to_bounding_box/1("vertex_a ")
  ScoutB_c/1 -> distance_to_bounding_box1/3(vertex_c)
  ScoutA_d/1 -> distance_to_bounding_box/4(vertex_d)
  CollectorB_c/1 -> distance_to_bounding_box2/3(vertex_c)
  ScoutA_b/1 -> distance_to_bounding_box/2(vertex_b)
  ScoutA_c/1 -> distance_to_bounding_box/3(vertex_c)
  origin_pos/1 -> distance_to_bounding_box2/5(sensor_pos), distance_to_bounding_box1/5(sensor_pos), distance_to_bounding_box/5(sensor_pos)
  Min/1 -> "distance_to_proximity_sensor_data "/1(distance_cm)
  sensor_ray_dir/1 -> distance_to_bounding_box2/6("sensor_ray "), distance_to_bounding_box1/6("sensor_ray "), distance_to_bounding_box/6("sensor_ray ")
  distance_to_bounding_box/1(distance) -> Min/1

== system boundingbox2/generate_proximity_sensor_readings/Subsystem2 ==
  origin_pos : Inport
  sensor_ray_dir : Inport  Port=2
  ScoutA_c : Inport  Port=3
  ScoutA_d : Inport  Port=4
  ScoutA_a : Inport  Port=5
  ScoutA_b : Inport  Port=6
  ScoutB_c : Inport  Port=7
  ScoutB_d : Inport  Port=8
  ScoutB_a : Inport  Port=9
  ScoutB_b : Inport  Port=10
  CollectorB_c : Inport  Port=11
  CollectorB_d : Inport  Port=12
  CollectorB_a : Inport  Port=13
  CollectorB_b : Inport  Port=14
  Min : MinMax  Inputs=3
  distance_to_bounding_box : Subsystem
  distance_to_bounding_box1 : Subsystem
  distance_to_bounding_box2 : Subsystem
  "distance_to_proximity_sensor_data " : Subsystem
  "sensor_data " : Outport
  wires:
  distance_to_bounding_box/1(distance) -> Min/1
  sensor_ray_dir/1 -> distance_to_bounding_box/6("sensor_ray "), distance_to_bounding_box1/6("sensor_ray "), distance_to_bounding_box2/6("sensor_ray ")
  Min/1 -> "distance_to_proximity_sensor_data "/1(distance_cm)
  origin_pos/1 -> distance_to_bounding_box/5(sensor_pos), distance_to_bounding_box1/5(sensor_pos), distance_to_bounding_box2/5(sensor_pos)
  ScoutA_c/1 -> distance_to_bounding_box/3(vertex_c)
  ScoutA_b/1 -> distance_to_bounding_box/2(vertex_b)
  CollectorB_c/1 -> distance_to_bounding_box2/3(vertex_c)
  ScoutA_d/1 -> distance_to_bounding_box/4(vertex_d)
  ScoutB_c/1 -> distance_to_bounding_box1/3(vertex_c)
  ScoutA_a/1 -> distance_to_bounding_box/1("vertex_a ")
  ScoutB_d/1 -> distance_to_bounding_box1/4(vertex_d)
  distance_to_bounding_box2/1(distance) -> Min/3
  ScoutB_b/1 -> distance_to_bounding_box1/2(vertex_b)
  ScoutB_a/1 -> distance_to_bounding_box1/1("vertex_a ")
  CollectorB_a/1 -> distance_to_bounding_box2/1("vertex_a ")
  CollectorB_d/1 -> distance_to_bounding_box2/4(vertex_d)
  distance_to_bounding_box1/1(distance) -> Min/2
  CollectorB_b/1 -> distance_to_bounding_box2/2(vertex_b)
  "distance_to_proximity_sensor_data "/1("prox_sensor_input ") -> "sensor_data "/1

== system boundingbox2/generate_proximity_sensor_readings/bounding_box_CollectorB ==
  note: output verteces of
      | bounding rectangle
      | C---D
      | |  >  |
      | B---A  as 2d vectors
  pos_x : Inport
  pos_y : Inport  Port=2
  theta : Inport  Port=3
  length : Inport  Port=4
  width : Inport  Port=5
  Add : Sum
  Add1 : Sum
  Gain : Gain  Gain=1/2
  Gain1 : Gain  Gain=1/2
  Gain2 : Gain  Gain=-1
  Subtract : Sum  Inputs=+-
  Subtract1 : Sum  Inputs=+-
  Vector Concatenate : Concatenate
  "vector rotation " : Subsystem
  vector rotation 1 : Subsystem
  vertex_a : Outport
  vertex_b : Outport  Port=2
  vertex_c : Outport  Port=3
  vertex_d : Outport  Port=4
  wires:
  Subtract1/1 -> vertex_d/1
  Add1/1 -> vertex_b/1
  Subtract/1 -> vertex_c/1
  Add/1 -> vertex_a/1
  vector rotation 1/1("rotated_vector ") -> Add1/2, Subtract1/2
  "vector rotation "/1("rotated_vector ") -> Add/2, Subtract/2
  Vector Concatenate/1 -> Add/1, Subtract/1, Add1/1, Subtract1/1
  Gain1/1 -> "vector rotation "/3(y_dir), vector rotation 1/3(y_dir)
  Gain2/1 -> vector rotation 1/2(x_dir)
  Gain/1 -> "vector rotation "/2(x_dir), Gain2/1
  theta/1 -> "vector rotation "/1(angle), vector rotation 1/1(angle)
  pos_y/1 -> Vector Concatenate/2
  pos_x/1 -> Vector Concatenate/1
  length/1 -> Gain/1
  width/1 -> Gain1/1

== system boundingbox2/generate_proximity_sensor_readings/bounding_box_ScoutA ==
  note: output verteces of
      | bounding rectangle
      | C---D
      | |  >  |
      | B---A  as 2d vectors
  pos_x : Inport
  pos_y : Inport  Port=2
  theta : Inport  Port=3
  length : Inport  Port=4
  width : Inport  Port=5
  Add : Sum
  Add1 : Sum
  Gain : Gain  Gain=1/2
  Gain1 : Gain  Gain=1/2
  Gain2 : Gain  Gain=-1
  Subtract : Sum  Inputs=+-
  Subtract1 : Sum  Inputs=+-
  Vector Concatenate : Concatenate
  "vector rotation " : Subsystem
  vector rotation 1 : Subsystem
  vertex_a : Outport
  vertex_b : Outport  Port=2
  vertex_c : Outport  Port=3
  vertex_d : Outport  Port=4
  wires:
  Subtract1/1 -> vertex_d/1
  Add1/1 -> vertex_b/1
  Subtract/1 -> vertex_c/1
  Add/1 -> vertex_a/1
  vector rotation 1/1("rotated_vector ") -> Add1/2, Subtract1/2
  "vector rotation "/1("rotated_vector ") -> Add/2, Subtract/2
  Vector Concatenate/1 -> Add/1, Subtract/1, Add1/1, Subtract1/1
  Gain1/1 -> "vector rotation "/3(y_dir), vector rotation 1/3(y_dir)
  Gain2/1 -> vector rotation 1/2(x_dir)
  Gain/1 -> "vector rotation "/2(x_dir), Gain2/1
  theta/1 -> "vector rotation "/1(angle), vector rotation 1/1(angle)
  pos_y/1 -> Vector Concatenate/2
  pos_x/1 -> Vector Concatenate/1
  length/1 -> Gain/1
  width/1 -> Gain1/1

== system boundingbox2/generate_proximity_sensor_readings/bounding_box_ScoutB ==
  note: output verteces of
      | bounding rectangle
      | C---D
      | |  >  |
      | B---A  as 2d vectors
  pos_x : Inport
  pos_y : Inport  Port=2
  theta : Inport  Port=3
  length : Inport  Port=4
  width : Inport  Port=5
  Add : Sum
  Add1 : Sum
  Gain : Gain  Gain=1/2
  Gain1 : Gain  Gain=1/2
  Gain2 : Gain  Gain=-1
  Subtract : Sum  Inputs=+-
  Subtract1 : Sum  Inputs=+-
  Vector Concatenate : Concatenate
  "vector rotation " : Subsystem
  vector rotation 1 : Subsystem
  vertex_a : Outport
  vertex_b : Outport  Port=2
  vertex_c : Outport  Port=3
  vertex_d : Outport  Port=4
  wires:
  width/1 -> Gain1/1
  length/1 -> Gain/1
  pos_x/1 -> Vector Concatenate/1
  pos_y/1 -> Vector Concatenate/2
  theta/1 -> vector rotation 1/1(angle), "vector rotation "/1(angle)
  Gain/1 -> Gain2/1, "vector rotation "/2(x_dir)
  Gain2/1 -> vector rotation 1/2(x_dir)
  Gain1/1 -> vector rotation 1/3(y_dir), "vector rotation "/3(y_dir)
  Vector Concatenate/1 -> Subtract1/1, Add1/1, Subtract/1, Add/1
  "vector rotation "/1("rotated_vector ") -> Subtract/2, Add/2
  vector rotation 1/1("rotated_vector ") -> Subtract1/2, Add1/2
  Add/1 -> vertex_a/1
  Subtract/1 -> vertex_c/1
  Add1/1 -> vertex_b/1
  Subtract1/1 -> vertex_d/1

== system boundingbox2/generate_proximity_sensor_readings/sensor_ray_generation front ==
  "theta " : Inport
  pos_x : Inport  Port=2
  pos_y : Inport  Port=3
  "sensor_dir (-1,0,1) " : Inport  Port=4
  Compare To Zero : simulink/Logic and Bit Operations/Compare To Zero  relop===  OutDataTypeStr=boolean
  Constant : Constant  Value=1.0
  Constant1 : Constant  Value=0
  Switch : Switch  Threshold=1
  Vector Concatenate : Concatenate
  "vector rotation " : Subsystem
  pos_2d : Outport
  "sensor_ray " : Outport  Port=2
  wires:
  "vector rotation "/1("rotated_vector ") -> "sensor_ray "/1
  pos_y/1 -> Vector Concatenate/2
  Vector Concatenate/1 -> pos_2d/1
  pos_x/1 -> Vector Concatenate/1
  "sensor_dir (-1,0,1) "/1 -> Compare To Zero/1, "vector rotation "/3(y_dir)
  "theta "/1 -> "vector rotation "/1(angle)
  Compare To Zero/1 -> Switch/2
  Constant/1 -> Switch/1
  Constant1/1 -> Switch/3
  Switch/1 -> "vector rotation "/2(x_dir)

== system boundingbox2/generate_proximity_sensor_readings/sensor_ray_generation left ==
  "theta " : Inport
  pos_x : Inport  Port=2
  pos_y : Inport  Port=3
  "sensor_dir (-1,0,1) " : Inport  Port=4
  Compare To Zero : simulink/Logic and Bit Operations/Compare To Zero  relop===  OutDataTypeStr=boolean
  Constant : Constant  Value=1.0
  Constant1 : Constant  Value=0
  Switch : Switch  Threshold=1
  Vector Concatenate : Concatenate
  "vector rotation " : Subsystem
  pos_2d : Outport
  "sensor_ray " : Outport  Port=2
  wires:
  Switch/1 -> "vector rotation "/2(x_dir)
  Constant1/1 -> Switch/3
  Constant/1 -> Switch/1
  Compare To Zero/1 -> Switch/2
  "theta "/1 -> "vector rotation "/1(angle)
  "sensor_dir (-1,0,1) "/1 -> "vector rotation "/3(y_dir), Compare To Zero/1
  pos_x/1 -> Vector Concatenate/1
  Vector Concatenate/1 -> pos_2d/1
  pos_y/1 -> Vector Concatenate/2
  "vector rotation "/1("rotated_vector ") -> "sensor_ray "/1

== system boundingbox2/generate_proximity_sensor_readings/sensor_ray_generation right ==
  "theta " : Inport
  pos_x : Inport  Port=2
  pos_y : Inport  Port=3
  "sensor_dir (-1,0,1) " : Inport  Port=4
  Compare To Zero : simulink/Logic and Bit Operations/Compare To Zero  relop===  OutDataTypeStr=boolean
  Constant : Constant  Value=1.0
  Constant1 : Constant  Value=0
  Switch : Switch  Threshold=1
  Vector Concatenate : Concatenate
  "vector rotation " : Subsystem
  pos_2d : Outport
  "sensor_ray " : Outport  Port=2
  wires:
  "vector rotation "/1("rotated_vector ") -> "sensor_ray "/1
  pos_y/1 -> Vector Concatenate/2
  Vector Concatenate/1 -> pos_2d/1
  pos_x/1 -> Vector Concatenate/1
  "sensor_dir (-1,0,1) "/1 -> Compare To Zero/1, "vector rotation "/3(y_dir)
  "theta "/1 -> "vector rotation "/1(angle)
  Compare To Zero/1 -> Switch/2
  Constant/1 -> Switch/1
  Constant1/1 -> Switch/3
  Switch/1 -> "vector rotation "/2(x_dir)

== system boundingbox2/sensor_ray_generation /vector rotation  ==
  angle : Inport
  x_dir : Inport  Port=2
  y_dir : Inport  Port=3
  Cos : Trigonometry  Operator=cos
  Multiply{,1..3} (4 alike) : Product
  Sin : Trigonometry
  Subtract : Sum  Inputs=+-
  Subtract1 : Sum
  Vector Concatenate1 : Concatenate
  "rotated_vector " : Outport
  wires:
  Multiply3/1 -> Subtract1/2
  Multiply1/1 -> Subtract1/1
  Multiply/1 -> Subtract/1
  y_dir/1 -> Multiply3/1, Multiply2/1
  Subtract1/1 -> Vector Concatenate1/2
  Cos/1 -> Multiply3/2, Multiply/2
  Sin/1 -> Multiply1/2, Multiply2/2
  angle/1 -> Cos/1, Sin/1
  x_dir/1 -> Multiply1/1, Multiply/1
  Vector Concatenate1/1 -> "rotated_vector "/1
  Subtract/1 -> Vector Concatenate1/1
  Multiply2/1 -> Subtract/2

== system boundingbox2/generate_proximity_sensor_readings/Subsystem/distance_to_bounding_box ==
  note: bounding rectangle
      | C---D
      | |  >  |
      | B---A
  "vertex_a " : Inport
  vertex_b : Inport  Port=2
  vertex_c : Inport  Port=3
  vertex_d : Inport  Port=4
  sensor_pos : Inport  Port=5
  "sensor_ray " : Inport  Port=6
  Inf{,1..3} (4 alike) : Constant  Value=inf
  Min : MinMax  Inputs=4
  Switch{,1..3} (4 alike) : Switch  Criteria=u2 > Threshold
  "calculate_intersection " : Subsystem
  calculate_intersection 1 : Subsystem
  calculate_intersection 2 : Subsystem
  calculate_intersection 3 : Subsystem
  distance : Outport
  wires:
  "vertex_a "/1 -> calculate_intersection 3/2(vertex_2), "calculate_intersection "/1(vertex_1)
  vertex_b/1 -> calculate_intersection 1/1(vertex_1), "calculate_intersection "/2(vertex_2)
  vertex_c/1 -> calculate_intersection 2/1(vertex_1), calculate_intersection 1/2(vertex_2)
  vertex_d/1 -> calculate_intersection 3/1(vertex_1), calculate_intersection 2/2(vertex_2)
  sensor_pos/1 -> calculate_intersection 3/3("origin "), calculate_intersection 2/3("origin "), calculate_intersection 1/3("origin "), "calculate_intersection "/3("origin ")
  "sensor_ray "/1 -> calculate_intersection 3/4(ray), calculate_intersection 2/4(ray), calculate_intersection 1/4(ray), "calculate_intersection "/4(ray)
  "calculate_intersection "/2(intersection (0,1)) -> Switch/2
  Inf/1 -> Switch/3
  Inf1/1 -> Switch1/3
  calculate_intersection 1/2(intersection (0,1)) -> Switch1/2
  calculate_intersection 2/2(intersection (0,1)) -> Switch2/2
  calculate_intersection 3/2(intersection (0,1)) -> Switch3/2
  Inf2/1 -> Switch2/3
  Inf3/1 -> Switch3/3
  calculate_intersection 3/1(distance) -> Switch3/1
  calculate_intersection 2/1(distance) -> Switch2/1
  calculate_intersection 1/1(distance) -> Switch1/1
  "calculate_intersection "/1(distance) -> Switch/1
  Switch/1 -> Min/1
  Switch1/1 -> Min/2
  Switch2/1 -> Min/3
  Switch3/1 -> Min/4
  Min/1 -> distance/1
